simulink model "simula_axebot_nao_linear_MPC"  (Simulink 8.5)
settings: Solver=ode3  StartTime=0.0  StopTime=6  FixedStep=0.05  MaxStep=0.01  RelTol=1e-6
values from neighbouring files (symbols this model uses):
  Ac = diag([(Ae-Bv)/M (Ae-Bvn)/M (Ae*b*b - Bw)/J])    [robo_MPC.m]
  Bc = [0 sqrt(3)/(2*M) -sqrt(3)/(2*M) ; -1/M 1/(2*M) 1/(2*M) ; b/J b/J b/J]*Be    [robo_MPC.m]
  deltaS = [deltaSv;deltaSvn;deltaSw]    [robo_MPC.m]
  Gc = Z    [robo_MPC.m]
  Kc = Z    [robo_MPC.m]
  ts = 0.06    [robo_MPC.m]
  Vnref = 0    [robo_MPC.m]
  Vref = 0.4    [robo_MPC.m]
  Vs = [Vsv;Vsvn;Vsw]    [robo_MPC.m]
  Wref = 0    [robo_MPC.m]
undefined symbols (not defined in the file or in its folder): Cd
settings Model: Creator=tito  LastModifiedBy=Jessivaldo
settings DebuggingCC: SolverPrmCheckMsg=warning  FcnCallInpInsideContextMsg=UseLocalSettings

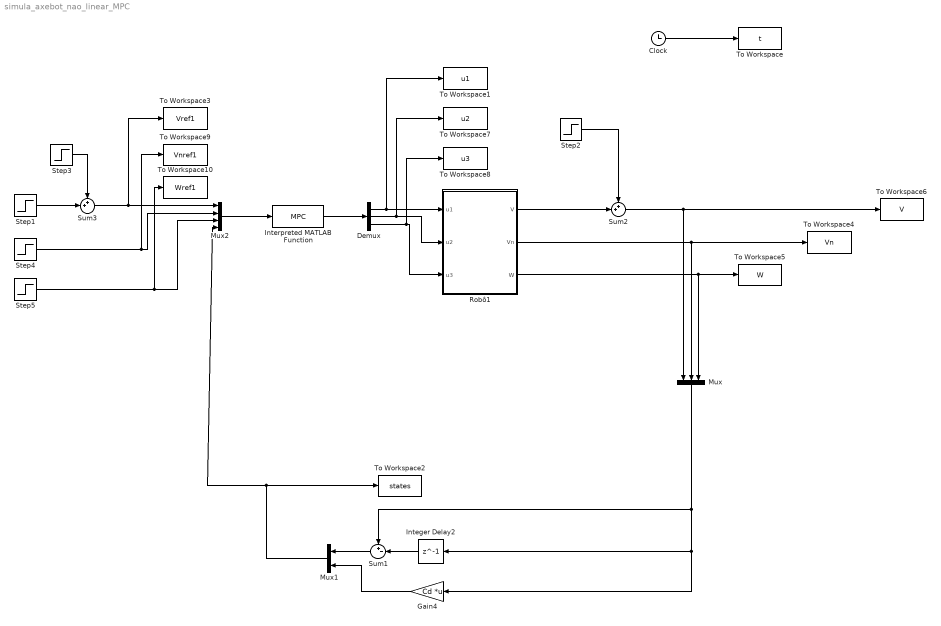
== system simula_axebot_nao_linear_MPC ==
  Clock : Clock
  Demux : Demux  Outputs=3
  Gain4 : Gain  Gain=Cd  Multiplication=Matrix(K*u)  SampleTime=ts
  Integer Delay2 : Delay  DelayLength=1  InputProcessing=Inherited  SampleTime=ts
  Interpreted MATLAB Function : MATLABFcn  MATLABFcn=MPC  OutputDimensions=3
  Mux : Mux  Inputs=3
  Mux1 : Mux  Inputs=2
  Mux2 : Mux
  Robô1 : Subsystem
  Step1 : Step  Time=0.5  After=Vref  SampleTime=ts
  Step2 : Step  Time=5  After=0.1*Vref  SampleTime=ts
  Step3 : Step  Time=2  After=-2*Vref  SampleTime=ts
  Step4 : Step  Time=0.5  After=Vnref  SampleTime=ts
  Step5 : Step  Time=0.5  After=Wref  SampleTime=ts
  Sum1 : Sum  Inputs=+-|
  Sum2 : Sum  Inputs=++|
  Sum3 : Sum  Inputs=++|
  To Workspace : ToWorkspace  VariableName=t  SampleTime=ts
  To Workspace1 : ToWorkspace  VariableName=u1  SampleTime=ts
  To Workspace10 : ToWorkspace  VariableName=Wref1  SampleTime=ts
  To Workspace2 : ToWorkspace  VariableName=states  SampleTime=ts
  To Workspace3 : ToWorkspace  VariableName=Vref1  SampleTime=ts
  To Workspace4 : ToWorkspace  VariableName=Vn  SampleTime=ts
  To Workspace5 : ToWorkspace  VariableName=W  SampleTime=ts
  To Workspace6 : ToWorkspace  VariableName=V  SampleTime=ts
  To Workspace7 : ToWorkspace  VariableName=u2  SampleTime=ts
  To Workspace8 : ToWorkspace  VariableName=u3  SampleTime=ts
  To Workspace9 : ToWorkspace  VariableName=Vnref1  SampleTime=ts
  wires:
  Clock/1 -> To Workspace/1
  Mux2/1 -> Interpreted MATLAB Function/1
  Sum1/1 -> Mux1/1
  Gain4/1 -> Mux1/2
  Integer Delay2/1 -> Sum1/2
  Mux1/1 -> Mux2/4, To Workspace2/1
  Robô1/1(V) -> Sum2/2
  Step2/1 -> Sum2/1
  Step1/1 -> Sum3/2
  Step3/1 -> Sum3/1
  Sum3/1 -> Mux2/1, To Workspace3/1
  Robô1/2(Vn) -> Mux/2, To Workspace4/1
  Robô1/3(W) -> Mux/3, To Workspace5/1
  Sum2/1 -> Mux/1, To Workspace6/1
  Mux/1 -> Gain4/1, Integer Delay2/1, Sum1/1
  Interpreted MATLAB Function/1 -> Demux/1
  Demux/1 -> Robô1/1(u1), To Workspace1/1
  Demux/2 -> To Workspace7/1, Robô1/2(u2)
  Demux/3 -> To Workspace8/1, Robô1/3(u3)
  Step4/1 -> To Workspace9/1, Mux2/2
  Step5/1 -> Mux2/3, To Workspace10/1

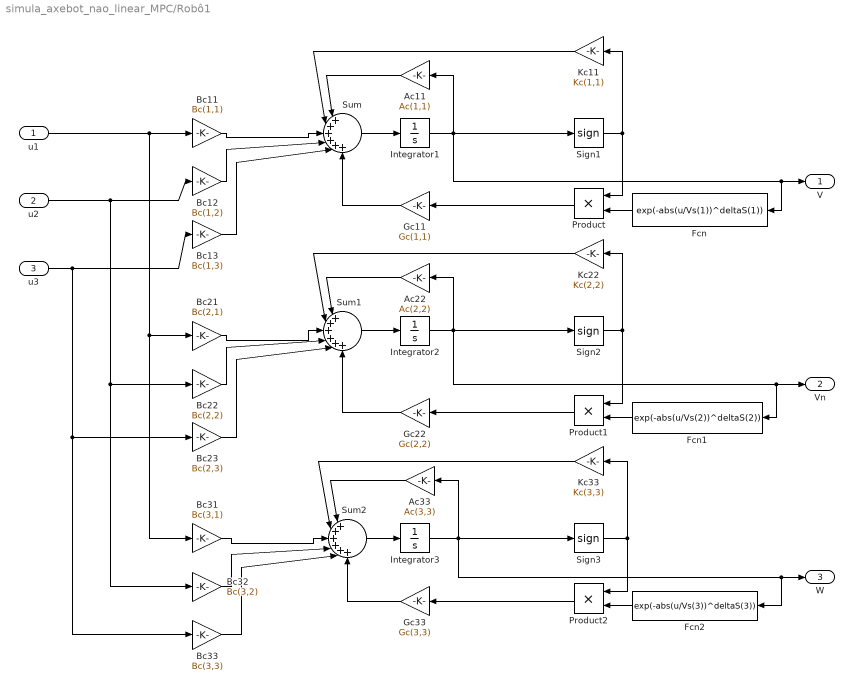
== system simula_axebot_nao_linear_MPC/Robô1 ==
  u1 : Inport
  u2 : Inport  Port=2
  u3 : Inport  Port=3
  Ac11 : Gain  Gain=Ac(1,1)
  Ac22 : Gain  Gain=Ac(2,2)
  Ac33 : Gain  Gain=Ac(3,3)
  Bc11 : Gain  Gain=Bc(1,1)
  Bc12 : Gain  Gain=Bc(1,2)
  Bc13 : Gain  Gain=Bc(1,3)
  Bc21 : Gain  Gain=Bc(2,1)
  Bc22 : Gain  Gain=Bc(2,2)
  Bc23 : Gain  Gain=Bc(2,3)
  Bc31 : Gain  Gain=Bc(3,1)
  Bc32 : Gain  Gain=Bc(3,2)
  Bc33 : Gain  Gain=Bc(3,3)
  Fcn : Fcn  Expr=exp(-abs(u/Vs(1))^deltaS(1))
  Fcn1 : Fcn  Expr=exp(-abs(u/Vs(2))^deltaS(2))
  Fcn2 : Fcn  Expr=exp(-abs(u/Vs(3))^deltaS(3))
  Gc11 : Gain  Gain=Gc(1,1)
  Gc22 : Gain  Gain=Gc(2,2)
  Gc33 : Gain  Gain=Gc(3,3)
  Integrator1 : Integrator
  Integrator2 : Integrator
  Integrator3 : Integrator
  Kc11 : Gain  Gain=Kc(1,1)
  Kc22 : Gain  Gain=Kc(2,2)
  Kc33 : Gain  Gain=Kc(3,3)
  Product : Product  RndMeth=Zero
  Product1 : Product  RndMeth=Zero
  Product2 : Product  RndMeth=Zero
  Sign1 : Signum  ZeroCross=off
  Sign2 : Signum  ZeroCross=off
  Sign3 : Signum  ZeroCross=off
  Sum : Sum  Inputs=|++++++
  Sum1 : Sum  Inputs=|++++++
  Sum2 : Sum  Inputs=|++++++
  V : Outport
  Vn : Outport  Port=2
  W : Outport  Port=3
  wires:
  Gc33/1 -> Sum2/6
  Gc22/1 -> Sum1/6
  Gc11/1 -> Sum/6
  Fcn2/1 -> Product2/2
  Fcn1/1 -> Product1/2
  Fcn/1 -> Product/2
  Kc33/1 -> Sum2/2
  Kc22/1 -> Sum1/2
  Kc11/1 -> Sum/2
  Product2/1 -> Gc33/1
  Product1/1 -> Gc22/1
  Product/1 -> Gc11/1
  Bc33/1 -> Sum2/5
  Bc32/1 -> Sum2/4
  Bc31/1 -> Sum2/3
  Sign3/1 -> Product2/1, Kc33/1
  Ac33/1 -> Sum2/1
  Integrator3/1 -> Fcn2/1, W/1, Sign3/1, Ac33/1
  Sum2/1 -> Integrator3/1
  Bc23/1 -> Sum1/5
  Bc22/1 -> Sum1/4
  Bc21/1 -> Sum1/3
  Sign2/1 -> Product1/1, Kc22/1
  Ac22/1 -> Sum1/1
  Integrator2/1 -> Fcn1/1, Vn/1, Sign2/1, Ac22/1
  Sum1/1 -> Integrator2/1
  Bc13/1 -> Sum/5
  Bc12/1 -> Sum/4
  Bc11/1 -> Sum/3
  Sign1/1 -> Product/1, Kc11/1
  Ac11/1 -> Sum/1
  Integrator1/1 -> Fcn/1, V/1, Sign1/1, Ac11/1
  Sum/1 -> Integrator1/1
  u3/1 -> Bc33/1, Bc23/1, Bc13/1
  u2/1 -> Bc32/1, Bc22/1, Bc12/1
  u1/1 -> Bc31/1, Bc21/1, Bc11/1
